simulink model "Despin_Simulink_Model"  (R2018a)
settings: Solver=VariableStepAuto  StartTime=0.0  StopTime=60  MaxStep=0.001  RelTol=1e-6  AbsTol=1e-6
values from neighbouring files (symbols this model uses):
  I_b = [151612935.5/10^9	       -12035.62/10^9        -9941.66/10^9 ... (first row only)    [Simulation_Parameters.m]
  I_single_rw = [220358.07/10^9         0               0 ... (first row only)    [Simulation_Parameters.m]
  I_st = [118601552.74/10^9	       -491524.85/10^9         95420.21/10^9 ... (first row only)    [Simulation_Parameters.m]
  m_b = 16.9927    [Simulation_Parameters.m]
  m_rw = 0.24806    [Simulation_Parameters.m]
  m_st = 9.48989    [Simulation_Parameters.m]
  R_0_to_1 = [sqrt(2)/2 0.5 0.5; -sqrt(2)/2 0.5 0.5; 0 -sqrt(2)/2 sqrt(2)/2]    [Simulation_Parameters.m]
undefined symbols (not defined in the file or in its folder): X, Y, Z
libraries: sm_lib x12, nesl_utility x10
settings Model: Creator=menel  LastModifiedBy=Menelaos
settings SolverCC: AlgebraicLoopSolver=LineSearch

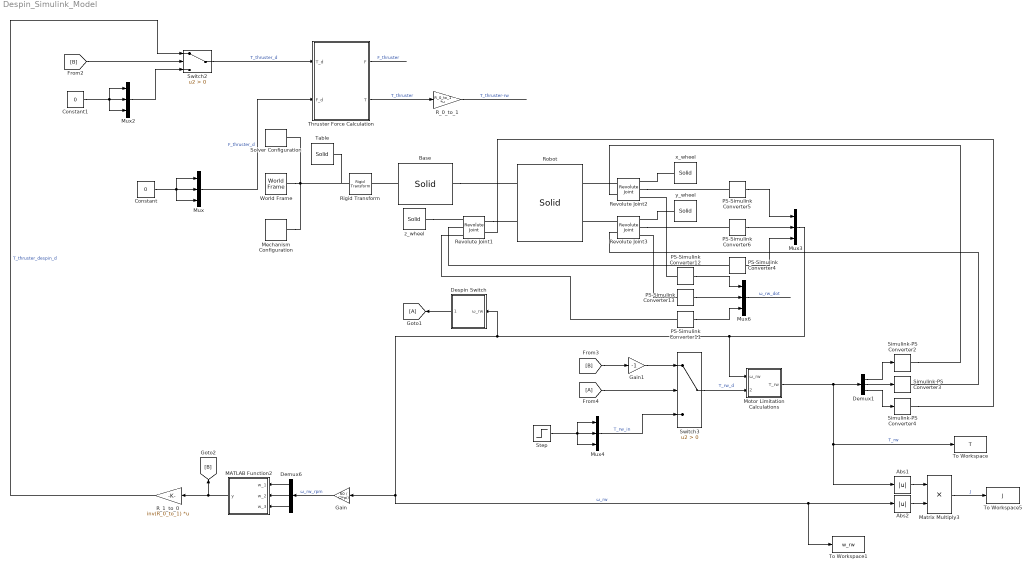
== system Despin_Simulink_Model ==
  Abs1 : Abs
  Abs2 : Abs
  Base : sm_lib/Body Elements/Solid  InertiaType=Custom  Mass=m_st  MassUnits=kg  CenterOfMass=COM_st  CenterOfMassUnits=m  MomentsOfInertia=[I_st(1,1) I_st(2,2) I_st(3,3)]  MomentsOfInertiaUnits=kg*m^2  ProductsOfInertia=[I_st(2,3) I_st(1,3) I_st(2,1)]  ProductsOfInertiaUnits=kg*m^2  DensityBased=on  Density=1000  DensityUnits=kg/m^3  DoExposeReferenceFrame=on  SerializedFrames=<Frames><Frame><Id>Frame1</Id><Value><Name>Rotation Frame</Name><Origin><Source>GeometricFeature</Source><FeatureName>spherical surface 1</FeatureName></Origin><PrimaryAxis><DefinedDirection>+Z</DefinedDirection><Source>ReferenceFrame</Source><SourceDirection>+Z</SourceDirection><FeatureName></FeatureName></PrimaryAxis><SecondaryAxis><DefinedDirection>+X</DefinedDirection><Source>ReferenceFrame</Source><SourceDirection>+X</SourceDirection><FeatureName></FeatureName></SecondaryAxis></Value></Frame></Frames>  GraphicType=FromGeometry  MarkerShape=Sphere  MarkerSize=10  GraphicVisPropType=SimpleVisualProperties  GraphicDiffuseColor=[1.0 0.2 0.2]  GraphicSpecularColor=[0.5 0.5 0.5 1.0]  GraphicAmbientColor=[0.15 0.15 0.15 1.0]  GraphicEmissiveColor=[0.0 0.0 0.0 1.0]  GraphicShininess=75  GraphicOpacity=1.0  GeometryShape=FromFile  RectangleSize=[1 1]  RectangleSizeUnits=m  BrickDimensions=[1 1 1]  BrickDimensionUnits=m  CylinderRadius=1  CylinderRadiusUnits=m  CylinderLength=1  CylinderLengthUnits=m  SphereRadius=1  SphereRadiusUnits=m  EllipsoidRadii=[1 1 1]  EllipsoidRadiiUnits=m  ExtrusionCrossSection=[1 1; -1 1; -1 -1; 1 -1]  ExtrusionCrossSectionUnits=m  ExtrusionLength=1  ExtrusionLengthUnits=m  PolygonNumSides=3  PolygonOuterRadius=1  PolygonOuterRadiusUnits=m  ExtGeomFileType=STEP  ExtGeomFileName=D:\School\Διπλωματική\Simulation\Simulation_13\Stand_6.STEP  ExtGeomFileUnits=m  RevolutionCrossSection=[1 1; 1 -1; 2 -1; 2 1]  RevolutionCrossSectionUnits=m  RevolutionExtent=Full  RevolutionAngle=180  RevolutionAngleUnits=deg
  Constant : Constant  Value=0
  Constant1 : Constant  Value=0
  Demux1 : Demux  Outputs=3
  Demux6 : Demux  Outputs=3
  Despin Switch : Subsystem
  Gain : Gain  Gain=60 / (2*pi)
  Gain1 : Gain  Gain=-1
  MATLAB Function2 : MATLAB Function  TreatAsAtomicUnit=on
  Matrix Multiply3 : Product
  Mechanism Configuration : sm_lib/Utilities/Mechanism Configuration  UniformGravity=Constant  GravityVector=[0 0 0]  GravityUnits=m/s^2  LinearizationDelta=0.001
  Motor Limitation Calculations : Subsystem
  Mux{,2..4,6} (5 alike) : Mux  Inputs=3
  PS-Simulink Converter11 : nesl_utility/PS-Simulink Converter  PhysicalDomain=network_engine_domain  SubClassName=ps_output  LeftPortType=input  RightPortType=output  PseudoPeriodic=off  Frequencies=[]  Unit=1  AffineConversion=off
  PS-Simulink Converter12 : nesl_utility/PS-Simulink Converter  PhysicalDomain=network_engine_domain  SubClassName=ps_output  LeftPortType=input  RightPortType=output  PseudoPeriodic=off  Frequencies=[]  Unit=1  AffineConversion=off
  PS-Simulink Converter13 : nesl_utility/PS-Simulink Converter  PhysicalDomain=network_engine_domain  SubClassName=ps_output  LeftPortType=input  RightPortType=output  PseudoPeriodic=off  Frequencies=[]  Unit=1  AffineConversion=off
  PS-Simulink Converter4 : nesl_utility/PS-Simulink Converter  PhysicalDomain=network_engine_domain  SubClassName=ps_output  LeftPortType=input  RightPortType=output  PseudoPeriodic=off  Frequencies=[]  Unit=rad/s  AffineConversion=off
  PS-Simulink Converter5 : nesl_utility/PS-Simulink Converter  PhysicalDomain=network_engine_domain  SubClassName=ps_output  LeftPortType=input  RightPortType=output  PseudoPeriodic=off  Frequencies=[]  Unit=rad/s  AffineConversion=off
  PS-Simulink Converter6 : nesl_utility/PS-Simulink Converter  PhysicalDomain=network_engine_domain  SubClassName=ps_output  LeftPortType=input  RightPortType=output  PseudoPeriodic=off  Frequencies=[]  Unit=rad/s  AffineConversion=off
  R_0_to_1 : Gain  Gain=R_0_to_1  Multiplication=Matrix(K*u) (u vector)
  R_1_to_0 : Gain  Gain=inv(R_0_to_1)  Multiplication=Matrix(K*u) (u vector)
  Revolute Joint1 : sm_lib/Joints/Revolute Joint  SenseConstraintForce=off  SenseConstraintForceX=off  SenseConstraintForceY=off  SenseConstraintForceZ=off  SenseConstraintTorque=off  SenseConstraintTorqueX=off  SenseConstraintTorqueY=off  SenseConstraintTorqueZ=off  SenseTotalForce=off  SenseTotalForceX=off  SenseTotalForceY=off  SenseTotalForceZ=off  SenseTotalTorque=off  SenseTotalTorqueX=off  SenseTotalTorqueY=off  SenseTotalTorqueZ=off  CompositeWrenchDir=FollowerOnBase  CompositeWrenchFrame=BaseFrame  EquilibriumPosition=0  EquilibriumPositionUnits=deg  SpringStiffness=0  SpringStiffnessUnits=N*m/deg  DampingCoefficient=0  DampingCoefficientUnits=N*m/(rad/s)  TorqueActuationMode=InputTorque  MotionActuationMode=ComputedMotion  SensePosition=off  SenseVelocity=on  SenseAcceleration=on  SenseTorqueForce=off  PositionTargetSpecify=on  PositionTargetPriority=High  PositionTargetValue=0  PositionTargetValueUnits=deg  VelocityTargetSpecify=off  VelocityTargetPriority=High  VelocityTargetValue=300  VelocityTargetValueUnits=rad/s
  Revolute Joint2 : sm_lib/Joints/Revolute Joint  SenseConstraintForce=off  SenseConstraintForceX=off  SenseConstraintForceY=off  SenseConstraintForceZ=off  SenseConstraintTorque=off  SenseConstraintTorqueX=off  SenseConstraintTorqueY=off  SenseConstraintTorqueZ=off  SenseTotalForce=off  SenseTotalForceX=off  SenseTotalForceY=off  SenseTotalForceZ=off  SenseTotalTorque=off  SenseTotalTorqueX=off  SenseTotalTorqueY=off  SenseTotalTorqueZ=off  CompositeWrenchDir=FollowerOnBase  CompositeWrenchFrame=BaseFrame  EquilibriumPosition=0  EquilibriumPositionUnits=deg  SpringStiffness=0  SpringStiffnessUnits=N*m/deg  DampingCoefficient=0  DampingCoefficientUnits=N*m/(rad/s)  TorqueActuationMode=InputTorque  MotionActuationMode=ComputedMotion  SensePosition=off  SenseVelocity=on  SenseAcceleration=on  SenseTorqueForce=off  PositionTargetSpecify=on  PositionTargetPriority=High  PositionTargetValue=0  PositionTargetValueUnits=deg  VelocityTargetSpecify=off  VelocityTargetPriority=High  VelocityTargetValue=300  VelocityTargetValueUnits=rad/s
  Revolute Joint3 : sm_lib/Joints/Revolute Joint  SenseConstraintForce=off  SenseConstraintForceX=off  SenseConstraintForceY=off  SenseConstraintForceZ=off  SenseConstraintTorque=off  SenseConstraintTorqueX=off  SenseConstraintTorqueY=off  SenseConstraintTorqueZ=off  SenseTotalForce=off  SenseTotalForceX=off  SenseTotalForceY=off  SenseTotalForceZ=off  SenseTotalTorque=off  SenseTotalTorqueX=off  SenseTotalTorqueY=off  SenseTotalTorqueZ=off  CompositeWrenchDir=FollowerOnBase  CompositeWrenchFrame=BaseFrame  EquilibriumPosition=0  EquilibriumPositionUnits=deg  SpringStiffness=0  SpringStiffnessUnits=N*m/deg  DampingCoefficient=0  DampingCoefficientUnits=N*m/(rad/s)  TorqueActuationMode=InputTorque  MotionActuationMode=ComputedMotion  SensePosition=off  SenseVelocity=on  SenseAcceleration=on  SenseTorqueForce=off  PositionTargetSpecify=on  PositionTargetPriority=High  PositionTargetValue=0  PositionTargetValueUnits=deg  VelocityTargetSpecify=off  VelocityTargetPriority=High  VelocityTargetValue=300  VelocityTargetValueUnits=rad/s
  Rigid Transform : sm_lib/Frames and Transforms/Rigid Transform  TranslationMethod=StandardAxis  TranslationStandardOffset=46  TranslationLengthUnit=mm  TranslationStandardAxis=+Z  TranslationCartesianOffset=[0 0 0]  TranslationROffset=0  TranslationROffsetUnits=m  TranslationZOffset=0  TranslationZOffsetUnits=m  TranslationThetaOffset=0  TranslationThetaOffsetUnits=deg  RotationMethod=None  RotationAngleUnits=deg  RotationStandardAxis=+Z  RotationAngle=0.0  RotationArbitraryAxis=[0 0 1]  FollAlignAxisA=+X  BaseAlignAxisA=+Y  FollAlignAxisB=+Y  BaseAlignAxisB=+Z  RotationSequenceAxes=FollowerAxes  RotationSequence=XYX  RotationSequenceAngles=[0 0 0]  RotationSequenceAnglesUnits=deg  RotationMatrix=[1 0 0; 0 1 0; 0 0 1]
  Robot : sm_lib/Body Elements/Solid  InertiaType=Custom  Mass=m_b  MassUnits=kg  CenterOfMass=COM_b  CenterOfMassUnits=m  MomentsOfInertia=[I_b(1,1) I_b(2,2) I_b(3,3)]  MomentsOfInertiaUnits=kg*m^2  ProductsOfInertia=[I_b(2,3) I_b(1,3) I_b(2,1)]  ProductsOfInertiaUnits=kg*m^2  DensityBased=off  Density=1000  DensityUnits=kg/m^3  DoExposeReferenceFrame=on  SerializedFrames=<Frames><Frame><Id>Frame1</Id><Value><Name>x wheel</Name><Origin><Source>GeometricFeature</Source><FeatureName>planar surface 30</FeatureName></Origin><PrimaryAxis><DefinedDirection>+Z</DefinedDirection><Source>GeometricFeature</Source><SourceDirection>+Z</SourceDirection><FeatureName>planar surface 30</FeatureName></PrimaryAxis><SecondaryAxis><DefinedDirection>+X</DefinedDirection><Source>ReferenceFrame</Source><SourceDirection>+X</SourceDirection><FeatureName></FeatureName></SecondaryAxis></Value></Frame><Frame><Id>Frame2</Id><Value><Name>y wheel</Name><Origin><Source>GeometricFeature</Source><FeatureName>planar surface 29</FeatureName></Origin><PrimaryAxis><DefinedDirection>+Z</DefinedDirection><Source>GeometricFeature</Source><SourceDirection>+Z</SourceDirection><FeatureName>planar surface 29</FeatureName></PrimaryAxis><SecondaryAxis><DefinedDirection>+X</DefinedDirection><Source>ReferenceFrame</Source><SourceDirection>+X</SourceDirection><FeatureName></FeatureName></SecondaryAxis></Value></Frame><Frame><Id>Frame3</Id><Value><Name>z wheel</Name><Origin><Source>GeometricFeature</Source><FeatureName>planar surface 31</FeatureName></Origin><PrimaryAxis><DefinedDirection>+Z</DefinedDirection><Source>GeometricFeature</Source><SourceDirection>+Z</SourceDirection><FeatureName>planar surface 31</FeatureName></PrimaryAxis><SecondaryAxis><DefinedDirection>+X</DefinedDirection><Source>ReferenceFrame</Source><SourceDirection>+X</SourceDirection><FeatureName></FeatureName></SecondaryAxis></Value></Frame></Frames>  GraphicType=FromGeometry  MarkerShape=Sphere  MarkerSize=10  GraphicVisPropType=SimpleVisualProperties  GraphicDiffuseColor=[0.6 0.6 1.0]  GraphicSpecularColor=[0.5 0.5 0.5 1.0]  GraphicAmbientColor=[0.15 0.15 0.15 1.0]  GraphicEmissiveColor=[0.0 0.0 0.0 1.0]  GraphicShininess=75  GraphicOpacity=1.0  GeometryShape=FromFile  RectangleSize=[1 1]  RectangleSizeUnits=m  BrickDimensions=[1 1 1]  BrickDimensionUnits=m  CylinderRadius=1  CylinderRadiusUnits=m  CylinderLength=1  CylinderLengthUnits=m  SphereRadius=1  SphereRadiusUnits=m  EllipsoidRadii=[1 1 1]  EllipsoidRadiiUnits=m  ExtrusionCrossSection=[1 1; -1 1; -1 -1; 1 -1]  ExtrusionCrossSectionUnits=m  ExtrusionLength=1  ExtrusionLengthUnits=m  PolygonNumSides=3  PolygonOuterRadius=1  PolygonOuterRadiusUnits=m  ExtGeomFileType=STEP  ExtGeomFileName=D:\School\Διπλωματική\Simulation\Simulation_13\Base_6.STEP  ExtGeomFileUnits=m  RevolutionCrossSection=[1 1; 1 -1; 2 -1; 2 1]  RevolutionCrossSectionUnits=m  RevolutionExtent=Full  RevolutionAngle=180  RevolutionAngleUnits=deg
  Simulink-PS Converter2 : nesl_utility/Simulink-PS Converter  PhysicalDomain=network_engine_domain  SubClassName=ps_input  LeftPortType=input  RightPortType=output  PseudoPeriodic=off  Frequencies=[]  NoiseDistribution=none  NoiseParameters=[]  Unit=N*m  AffineConversion=off  FilteringAndDerivatives=zero  SimscapeFilterOrder=1  InputFilterTimeConstant=0.001  UdotUserProvided=1
  Simulink-PS Converter3 : nesl_utility/Simulink-PS Converter  PhysicalDomain=network_engine_domain  SubClassName=ps_input  LeftPortType=input  RightPortType=output  PseudoPeriodic=off  Frequencies=[]  NoiseDistribution=none  NoiseParameters=[]  Unit=N*m  AffineConversion=off  FilteringAndDerivatives=zero  SimscapeFilterOrder=1  InputFilterTimeConstant=0.001  UdotUserProvided=1
  Simulink-PS Converter4 : nesl_utility/Simulink-PS Converter  PhysicalDomain=network_engine_domain  SubClassName=ps_input  LeftPortType=input  RightPortType=output  PseudoPeriodic=off  Frequencies=[]  NoiseDistribution=none  NoiseParameters=[]  Unit=N*m  AffineConversion=off  FilteringAndDerivatives=zero  SimscapeFilterOrder=1  InputFilterTimeConstant=0.001  UdotUserProvided=1
  Solver Configuration : nesl_utility/Solver Configuration  PhysicalDomain=network_engine_domain  SubClassName=solver  LeftPortType=input  RightPortType=generic  Tones=[]  Harmonics=[]  SimulateNoise=off  Profile=off  UseLocalSampling=off  EnableSwitchedLinearOptims=on  FrequencyDomain=off  UseCCode=off  RelTol=0.001  AbsTol=1e-06  MinStep=1e-09  ToWorkspace=off  RevertToSquareIcSolve=off  NumHomotopyIterations=100  PhasorMode=off  PhasorModeNumHarmonics=1  DoDC=off  ResidualTolerance=1e-09  UseLocalSolver=off  LocalSolverChoice=NE_BACKWARD_EULER_ADVANCER  LocalSolverSampleTime=0.001  DoFixedCost=off  MaxNonlinIter=3  MaxModeIter=2  LinearAlgebra=Sparse  EquationFormulation=NE_TIME_EF  DelaysMemoryBudget=1024  AutomaticFiltering=on  FilteringTimeConstant=0.001
  Step : Step  Time=30  Before=0.01  After=0  SampleTime=0
  Switch2 : Switch  Criteria=u2 > Threshold
  Switch3 : Switch  Criteria=u2 > Threshold
  Table : sm_lib/Body Elements/Solid  InertiaType=CalculateFromGeometry  Mass=1  MassUnits=kg  CenterOfMass=[0 0 0]  CenterOfMassUnits=m  MomentsOfInertia=[1 1 1]  MomentsOfInertiaUnits=kg*m^2  ProductsOfInertia=[0 0 0]  ProductsOfInertiaUnits=kg*m^2  DensityBased=on  Density=1000  DensityUnits=kg/m^3  DoExposeReferenceFrame=on  SerializedFrames=<Frames/>  GraphicType=FromGeometry  MarkerShape=Sphere  MarkerSize=10  GraphicVisPropType=SimpleVisualProperties  GraphicDiffuseColor=[0.5 0.5 0.5]  GraphicSpecularColor=[0.5 0.5 0.5 1.0]  GraphicAmbientColor=[0.15 0.15 0.15 1.0]  GraphicEmissiveColor=[0.0 0.0 0.0 1.0]  GraphicShininess=75  GraphicOpacity=1.0  GeometryShape=FromFile  RectangleSize=[1 1]  RectangleSizeUnits=m  BrickDimensions=[1 1 1]  BrickDimensionUnits=m  CylinderRadius=1  CylinderRadiusUnits=m  CylinderLength=1  CylinderLengthUnits=m  SphereRadius=1  SphereRadiusUnits=m  EllipsoidRadii=[1 1 1]  EllipsoidRadiiUnits=m  ExtrusionCrossSection=[1 1; -1 1; -1 -1; 1 -1]  ExtrusionCrossSectionUnits=m  ExtrusionLength=1  ExtrusionLengthUnits=m  PolygonNumSides=3  PolygonOuterRadius=1  PolygonOuterRadiusUnits=m  ExtGeomFileType=STEP  ExtGeomFileName=D:\School\Διπλωματική\Simulation\Simulation_13\Table.STEP  ExtGeomFileUnits=m  RevolutionCrossSection=[1 1; 1 -1; 2 -1; 2 1]  RevolutionCrossSectionUnits=m  RevolutionExtent=Full  RevolutionAngle=180  RevolutionAngleUnits=deg
  Thruster Force Calculation : Subsystem
  To Workspace : ToWorkspace  VariableName=T  SampleTime=-1
  To Workspace1 : ToWorkspace  VariableName=w_rw  SampleTime=-1
  To Workspace5 : ToWorkspace  VariableName=J  SampleTime=-1
  World Frame : sm_lib/Frames and Transforms/World Frame
  x_wheel : sm_lib/Body Elements/Solid  InertiaType=Custom  Mass=m_rw  MassUnits=kg  CenterOfMass=COM_rw  CenterOfMassUnits=m  MomentsOfInertia=[I_single_rw(1,1) I_single_rw(2,2) I_single_rw(3,3)]  MomentsOfInertiaUnits=kg*m^2  ProductsOfInertia=[I_single_rw(2,3) I_single_rw(1,3) I_single_rw(2,1)]  ProductsOfInertiaUnits=kg*m^2  DensityBased=off  Density=1000  DensityUnits=kg/m^3  DoExposeReferenceFrame=off  SerializedFrames=<Frames><Frame><Id>Frame1</Id><Value><Name>R</Name><Origin><Source>GeometricFeature</Source><FeatureName>planar surface 2</FeatureName></Origin><PrimaryAxis><DefinedDirection>+Z</DefinedDirection><Source>ReferenceFrame</Source><SourceDirection>+Z</SourceDirection><FeatureName></FeatureName></PrimaryAxis><SecondaryAxis><DefinedDirection>+X</DefinedDirection><Source>ReferenceFrame</Source><SourceDirection>+X</SourceDirection><FeatureName></FeatureName></SecondaryAxis></Value></Frame></Frames>  GraphicType=FromGeometry  MarkerShape=Sphere  MarkerSize=10  GraphicVisPropType=SimpleVisualProperties  GraphicDiffuseColor=[1.0 0.2 0.2]  GraphicSpecularColor=[0.5 0.5 0.5 1.0]  GraphicAmbientColor=[0.15 0.15 0.15 1.0]  GraphicEmissiveColor=[0.0 0.0 0.0 1.0]  GraphicShininess=75  GraphicOpacity=1.0  GeometryShape=FromFile  RectangleSize=[1 1]  RectangleSizeUnits=m  BrickDimensions=[1 1 1]  BrickDimensionUnits=m  CylinderRadius=1  CylinderRadiusUnits=m  CylinderLength=1  CylinderLengthUnits=m  SphereRadius=1  SphereRadiusUnits=m  EllipsoidRadii=[1 1 1]  EllipsoidRadiiUnits=m  ExtrusionCrossSection=[1 1; -1 1; -1 -1; 1 -1]  ExtrusionCrossSectionUnits=m  ExtrusionLength=1  ExtrusionLengthUnits=m  PolygonNumSides=3  PolygonOuterRadius=1  PolygonOuterRadiusUnits=m  ExtGeomFileType=STEP  ExtGeomFileName=D:\School\Διπλωματική\Simulation\Simulation_13\Reaction_Wheel_6.STEP  ExtGeomFileUnits=m  RevolutionCrossSection=[1 1; 1 -1; 2 -1; 2 1]  RevolutionCrossSectionUnits=m  RevolutionExtent=Full  RevolutionAngle=180  RevolutionAngleUnits=deg
  y_wheel : sm_lib/Body Elements/Solid  InertiaType=Custom  Mass=m_rw  MassUnits=kg  CenterOfMass=COM_rw  CenterOfMassUnits=m  MomentsOfInertia=[I_single_rw(1,1) I_single_rw(2,2) I_single_rw(3,3)]  MomentsOfInertiaUnits=kg*m^2  ProductsOfInertia=[I_single_rw(2,3) I_single_rw(1,3) I_single_rw(2,1)]  ProductsOfInertiaUnits=kg*m^2  DensityBased=off  Density=1000  DensityUnits=kg/m^3  DoExposeReferenceFrame=off  SerializedFrames=<Frames><Frame><Id>Frame1</Id><Value><Name>R</Name><Origin><Source>GeometricFeature</Source><FeatureName>planar surface 2</FeatureName></Origin><PrimaryAxis><DefinedDirection>+Z</DefinedDirection><Source>ReferenceFrame</Source><SourceDirection>+Z</SourceDirection><FeatureName></FeatureName></PrimaryAxis><SecondaryAxis><DefinedDirection>+X</DefinedDirection><Source>ReferenceFrame</Source><SourceDirection>+X</SourceDirection><FeatureName></FeatureName></SecondaryAxis></Value></Frame></Frames>  GraphicType=FromGeometry  MarkerShape=Sphere  MarkerSize=10  GraphicVisPropType=SimpleVisualProperties  GraphicDiffuseColor=[1.0 0.2 0.2]  GraphicSpecularColor=[0.5 0.5 0.5 1.0]  GraphicAmbientColor=[0.15 0.15 0.15 1.0]  GraphicEmissiveColor=[0.0 0.0 0.0 1.0]  GraphicShininess=75  GraphicOpacity=1.0  GeometryShape=FromFile  RectangleSize=[1 1]  RectangleSizeUnits=m  BrickDimensions=[1 1 1]  BrickDimensionUnits=m  CylinderRadius=1  CylinderRadiusUnits=m  CylinderLength=1  CylinderLengthUnits=m  SphereRadius=1  SphereRadiusUnits=m  EllipsoidRadii=[1 1 1]  EllipsoidRadiiUnits=m  ExtrusionCrossSection=[1 1; -1 1; -1 -1; 1 -1]  ExtrusionCrossSectionUnits=m  ExtrusionLength=1  ExtrusionLengthUnits=m  PolygonNumSides=3  PolygonOuterRadius=1  PolygonOuterRadiusUnits=m  ExtGeomFileType=STEP  ExtGeomFileName=D:\School\Διπλωματική\Simulation\Simulation_13\Reaction_Wheel_6.STEP  ExtGeomFileUnits=m  RevolutionCrossSection=[1 1; 1 -1; 2 -1; 2 1]  RevolutionCrossSectionUnits=m  RevolutionExtent=Full  RevolutionAngle=180  RevolutionAngleUnits=deg
  z_wheel : sm_lib/Body Elements/Solid  InertiaType=Custom  Mass=m_rw  MassUnits=kg  CenterOfMass=COM_rw  CenterOfMassUnits=m  MomentsOfInertia=[I_single_rw(1,1) I_single_rw(2,2) I_single_rw(3,3)]  MomentsOfInertiaUnits=kg*m^2  ProductsOfInertia=[I_single_rw(2,3) I_single_rw(1,3) I_single_rw(2,1)]  ProductsOfInertiaUnits=kg*m^2  DensityBased=off  Density=1000  DensityUnits=kg/m^3  DoExposeReferenceFrame=off  SerializedFrames=<Frames><Frame><Id>Frame1</Id><Value><Name>R</Name><Origin><Source>GeometricFeature</Source><FeatureName>planar surface 2</FeatureName></Origin><PrimaryAxis><DefinedDirection>+Z</DefinedDirection><Source>ReferenceFrame</Source><SourceDirection>+Z</SourceDirection><FeatureName></FeatureName></PrimaryAxis><SecondaryAxis><DefinedDirection>+X</DefinedDirection><Source>ReferenceFrame</Source><SourceDirection>+X</SourceDirection><FeatureName></FeatureName></SecondaryAxis></Value></Frame></Frames>  GraphicType=FromGeometry  MarkerShape=Sphere  MarkerSize=10  GraphicVisPropType=SimpleVisualProperties  GraphicDiffuseColor=[1.0 0.2 0.2]  GraphicSpecularColor=[0.5 0.5 0.5 1.0]  GraphicAmbientColor=[0.15 0.15 0.15 1.0]  GraphicEmissiveColor=[0.0 0.0 0.0 1.0]  GraphicShininess=75  GraphicOpacity=1.0  GeometryShape=FromFile  RectangleSize=[1 1]  RectangleSizeUnits=m  BrickDimensions=[1 1 1]  BrickDimensionUnits=m  CylinderRadius=1  CylinderRadiusUnits=m  CylinderLength=1  CylinderLengthUnits=m  SphereRadius=1  SphereRadiusUnits=m  EllipsoidRadii=[1 1 1]  EllipsoidRadiiUnits=m  ExtrusionCrossSection=[1 1; -1 1; -1 -1; 1 -1]  ExtrusionCrossSectionUnits=m  ExtrusionLength=1  ExtrusionLengthUnits=m  PolygonNumSides=3  PolygonOuterRadius=1  PolygonOuterRadiusUnits=m  ExtGeomFileType=STEP  ExtGeomFileName=D:\School\Διπλωματική\Simulation\Simulation_13\Reaction_Wheel_6.STEP  ExtGeomFileUnits=m  RevolutionCrossSection=[1 1; 1 -1; 2 -1; 2 1]  RevolutionCrossSectionUnits=m  RevolutionExtent=Full  RevolutionAngle=180  RevolutionAngleUnits=deg
  wires:
  Mux/1 -> Thruster Force Calculation/2(F_d)  "F_thruster_d"
  Thruster Force Calculation/1(F) -> ?  "F_thruster"
  Thruster Force Calculation/2(T) -> R_0_to_1/1  "T_thruster"
  PS-Simulink Converter6/1 -> Mux3/2
  PS-Simulink Converter5/1 -> Mux3/1
  PS-Simulink Converter4/1 -> Mux3/3
  Mux3/1 -> Motor Limitation Calculations/1(ω_rw), To Workspace1/1, Abs2/1, Gain/1, Despin Switch/1(ω_rw)  "ω_rw"
  Demux1/2 -> Simulink-PS Converter3/1
  Demux1/3 -> Simulink-PS Converter4/1
  Demux1/1 -> Simulink-PS Converter2/1
  Mux6/1 -> ?  "ω_rw_dot"
  Constant/1 -> Mux/3, Mux/1, Mux/2
  PS-Simulink Converter12/1 -> Mux6/1
  PS-Simulink Converter13/1 -> Mux6/2
  PS-Simulink Converter11/1 -> Mux6/3
  Gain/1 -> Demux6/1  "ω_rw_rpm"
  Demux6/3 -> MATLAB Function2/3(w_3)
  Demux6/2 -> MATLAB Function2/2(w_2)
  Demux6/1 -> MATLAB Function2/1(w_1)
  MATLAB Function2/1(y) -> [B], R_1_to_0/1
  [B] -> Switch2/2
  Switch2/1 -> Thruster Force Calculation/1(T_d)  "T_thruster_d"
  Mux2/1 -> Switch2/3
  Constant1/1 -> Mux2/3, Mux2/1, Mux2/2
  R_0_to_1/1 -> ?  "T_thruster-rw"
  R_1_to_0/1 -> Switch2/1  "T_thruster_despin_d"
  [A] -> Switch3/2
  Mux4/1 -> Switch3/3  "T_rw_in"
  [B] -> Gain1/1
  Despin Switch/1(signal) -> [A]
  Step/1 -> Mux4/3, Mux4/1, Mux4/2
  Motor Limitation Calculations/1(T_rw) -> To Workspace/1, Abs1/1, Demux1/1  "T_rw"
  Switch3/1 -> Motor Limitation Calculations/2(T_rw_d)  "T_rw_d"
  Gain1/1 -> Switch3/1
  Abs2/1 -> Matrix Multiply3/2
  Abs1/1 -> Matrix Multiply3/1
  Matrix Multiply3/1 -> To Workspace5/1  "J"
  connections:
  World Frame/RConn1 -- Mechanism Configuration/RConn1 -- Table/RConn1 -- Rigid Transform/LConn1 -- Solver Configuration/RConn1
  Base/RConn1 -- Rigid Transform/RConn1
  Revolute Joint1/LConn1 -- Robot/RConn2
  z_wheel/LConn1 -- Revolute Joint1/RConn1
  Revolute Joint2/LConn1 -- Robot/LConn1
  Revolute Joint3/LConn1 -- Robot/LConn2
  x_wheel/LConn1 -- Revolute Joint2/RConn1
  y_wheel/LConn1 -- Revolute Joint3/RConn1
  Revolute Joint2/RConn2 -- PS-Simulink Converter5/LConn1
  Revolute Joint3/RConn2 -- PS-Simulink Converter6/LConn1
  PS-Simulink Converter4/LConn1 -- Revolute Joint1/RConn2
  Simulink-PS Converter2/RConn1 -- Revolute Joint2/LConn2
  Simulink-PS Converter3/RConn1 -- Revolute Joint3/LConn2
  Simulink-PS Converter4/RConn1 -- Revolute Joint1/LConn2
  PS-Simulink Converter12/LConn1 -- Revolute Joint2/RConn3
  PS-Simulink Converter13/LConn1 -- Revolute Joint3/RConn3
  PS-Simulink Converter11/LConn1 -- Revolute Joint1/RConn3
  Base/LConn1 -- Robot/RConn1

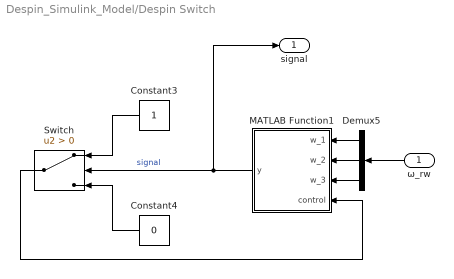
== system Despin_Simulink_Model/Despin Switch ==
  ω_rw : Inport
  Constant3 : Constant
  Constant4 : Constant  Value=0
  Demux5 : Demux  Outputs=3
  MATLAB Function1 : MATLAB Function  TreatAsAtomicUnit=on
  Switch : Switch  Criteria=u2 > Threshold
  signal : Outport
  wires:
  ω_rw/1 -> Demux5/1
  Demux5/3 -> MATLAB Function1/3(w_3)
  Demux5/1 -> MATLAB Function1/1(w_1)
  Constant3/1 -> Switch/1
  Switch/1 -> MATLAB Function1/4(control)
  MATLAB Function1/1(y) -> signal/1, Switch/2  "signal"
  Constant4/1 -> Switch/3
  Demux5/2 -> MATLAB Function1/2(w_2)

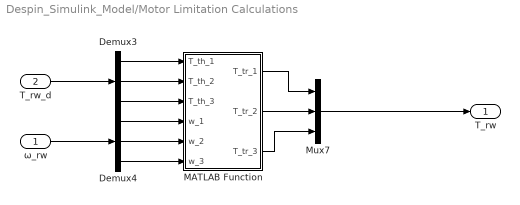
== system Despin_Simulink_Model/Motor Limitation Calculations ==
  ω_rw : Inport
  T_rw_d : Inport  Port=2
  Demux3 : Demux  Outputs=3
  Demux4 : Demux  Outputs=3
  MATLAB Function : MATLAB Function  TreatAsAtomicUnit=on
  Mux7 : Mux  Inputs=3
  T_rw : Outport
  wires:
  Demux3/1 -> MATLAB Function/1(T_th_1)
  Demux4/1 -> MATLAB Function/4(w_1)
  Demux3/3 -> MATLAB Function/3(T_th_3)
  Demux4/2 -> MATLAB Function/5(w_2)
  MATLAB Function/3(T_tr_3) -> Mux7/3
  Demux3/2 -> MATLAB Function/2(T_th_2)
  MATLAB Function/2(T_tr_2) -> Mux7/2
  MATLAB Function/1(T_tr_1) -> Mux7/1
  Demux4/3 -> MATLAB Function/6(w_3)
  ω_rw/1 -> Demux4/1
  Mux7/1 -> T_rw/1
  T_rw_d/1 -> Demux3/1

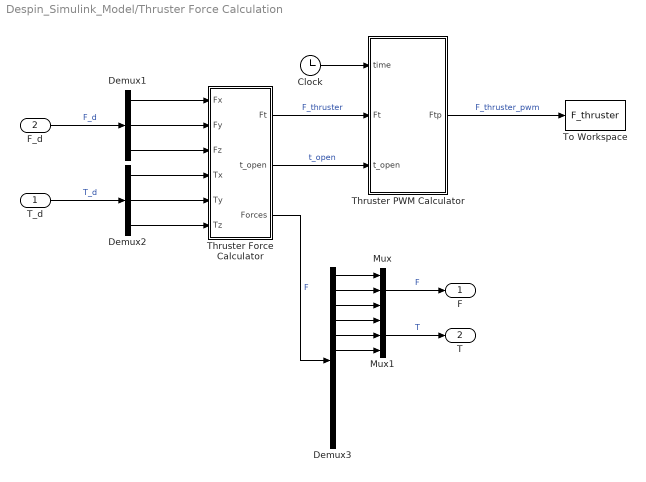
== system Despin_Simulink_Model/Thruster Force Calculation ==
  T_d : Inport
  F_d : Inport  Port=2
  Clock : Clock
  Demux1 : Demux  Outputs=3
  Demux2 : Demux  Outputs=3
  Demux3 : Demux  Outputs=12
  Mux : Mux  Inputs=3
  Mux1 : Mux  Inputs=3
  Thruster Force Calculator : MATLAB Function  TreatAsAtomicUnit=on
  Thruster PWM Calculator : MATLAB Function  TreatAsAtomicUnit=on
  To Workspace : ToWorkspace  VariableName=F_thruster  SampleTime=-1
  F : Outport
  T : Outport  Port=2
  wires:
  Demux2/3 -> Thruster Force Calculator/6(Tz)
  Demux1/3 -> Thruster Force Calculator/3(Fz)
  Demux2/1 -> Thruster Force Calculator/4(Tx)
  Demux1/2 -> Thruster Force Calculator/2(Fy)
  Demux1/1 -> Thruster Force Calculator/1(Fx)
  Demux2/2 -> Thruster Force Calculator/5(Ty)
  T_d/1 -> Demux2/1  "T_d"
  F_d/1 -> Demux1/1  "F_d"
  Thruster Force Calculator/2(t_open) -> Thruster PWM Calculator/3(t_open)  "t_open"
  Thruster Force Calculator/1(Ft) -> Thruster PWM Calculator/2(Ft)  "F_thruster"
  Clock/1 -> Thruster PWM Calculator/1(time)
  Thruster PWM Calculator/1(Ftp) -> To Workspace/1  "F_thruster_pwm"
  Thruster Force Calculator/3(Forces) -> Demux3/1  "F"
  Demux3/1 -> Mux/1
  Demux3/2 -> Mux/2
  Demux3/3 -> Mux/3
  Demux3/4 -> Mux1/1
  Demux3/5 -> Mux1/2
  Demux3/6 -> Mux1/3
  Mux/1 -> F/1  "F"
  Mux1/1 -> T/1  "T"

== matlab function Despin_Simulink_Model/Thruster Force Calculation/Thruster Force Calculator ==
  data: Ft output; t_open output; Fx input; Fy input; Fz input; Tx input; Ty input; Tz input; Forces output
function [Ft,t_open,Forces]= fcn(Fx,Fy,Fz,Tx,Ty,Tz)

f = [Fx;Fy;Fz;Tx;Ty;Tz];

d = 0.2335;
T = 0.1;

A = [-1  cosd(60)   cosd(60)  0        0            0;
      0  sind(60)  -sind(60)  0        0            0;
      0     0          0      1        1            1;
      0     0          0      d  -d*cosd(30)  -d*cosd(30);
      0     0          0      0  -d*sind(30)   d*sind(30);
      d     d          d      0        0            0   ];

Ft_d = inv(A)*f;

Ft = [0;0;0;0;0;0;0;0;0;0;0;0];
t_open = [0;0;0;0;0;0;0;0;0;0;0;0];

if Ft_d(1) == 0
    
    Ft(1) = 0;
    Ft(2) = 0;
    t_open(1) = 0;
    t_open(2) = 0;
    
elseif Ft_d(1) > 0
    
    Ft(1) = 1;
    Ft(2) = 0;
    t_open(1) = abs(Ft_d(1)*T);
    t_open(2) = 0;
    
else
    
    Ft(1) = 0;
    Ft(2) = 1;
    t_open(1) = 0;
    t_open(2) = abs(Ft_d(1)*T);
    
end

%%%%%%%%%%%%%%%%%%%%%%%%%%%%%%%%%%%%%%%%%%%%%%%%%%%%%%%%%%%%%%

if Ft_d(2) == 0
    
    Ft(3) = 0;
    Ft(4) = 0;
    t_open(3) = 0;
    t_open(4) = 0;
    
elseif Ft_d(2) > 0
    
    Ft(3) = 1;
    Ft(4) = 0;
    t_open(3) = abs(Ft_d(2)*T);
    t_open(4) = 0;
    
else
    
    Ft(3) = 0;
    Ft(4) = 1;
    t_open(3) = 0;
    t_open(4) = abs(Ft_d(2)*T);
    
end

%%%%%%%%%%%%%%%%%%%%%%%%%%%%%%%%%%%%%%%%%%%%%%%%%%%%%%%%%%%%%%

if Ft_d(3) == 0
    
    Ft(5) = 0;
    Ft(6) = 0;
    t_open(5) = 0;
    t_open(6) = 0;
    
elseif Ft_d(3) > 0
    
    Ft(5) = 1;
    Ft(6) = 0;
    t_open(5) = abs(Ft_d(3)*T);
    t_open(6) = 0;
    
else
    
    Ft(5) = 0;
    Ft(6) = 1;
    t_open(5) = 0;
    t_open(6) = abs(Ft_d(3)*T);
    
end

%%%%%%%%%%%%%%%%%%%%%%%%%%%%%%%%%%%%%%%%%%%%%%%%%%%%%%%%%%%%%%

if Ft_d(4) == 0
    
    Ft(7) = 0;
    Ft(8) = 0;
    t_open(7) = 0;
    t_open(8) = 0;
    
elseif Ft_d(4) > 0
    
    Ft(7) = 1;
    Ft(8) = 0;
    t_open(7) = abs(Ft_d(4)*T);
    t_open(8) = 0;
    
else
    
    Ft(7) = 0;
    Ft(8) = 1;
    t_open(7) = 0;
    t_open(8) = abs(Ft_d(4)*T);
    
end

%%%%%%%%%%%%%%%%%%%%%%%%%%%%%%%%%%%%%%%%%%%%%%%%%%%%%%%%%%%%%%

if Ft_d(5) == 0
    
    Ft(9) = 0;
    Ft(10) = 0;
    t_open(9) = 0;
    t_open(10) = 0;
    
elseif Ft_d(5) > 0
    
    Ft(9) = 1;
    Ft(10) = 0;
    t_open(9) = abs(Ft_d(5)*T);
    t_open(10) = 0;
    
else
    
    Ft(9) = 0;
    Ft(10) = 1;
    t_open(9) = 0;
    t_open(10) = abs(Ft_d(5)*T);
    
end

%%%%%%%%%%%%%%%%%%%%%%%%%%%%%%%%%%%%%%%%%%%%%%%%%%%%%%%%%%%%%%

if Ft_d(6) == 0
    
    Ft(11) = 0;
    Ft(12) = 0;
    t_open(11) = 0;
    t_open(12) = 0;
    
elseif Ft_d(6) > 0
    
    Ft(11) = 1;
    Ft(12) = 0;
    t_open(11) = abs(Ft_d(6)*T);
    t_open(12) = 0;
    
else
    
    Ft(11) = 0;
    Ft(12) = 1;
    t_open(11) = 0;
    t_open(12) = abs(Ft_d(6)*T);
    
end

for i = 1:6
    if Ft_d(i) > 1
        
        Ft_d(i) = 1;
        
    elseif Ft_d(i) < -1
        
        Ft_d(i) = -1;
        
    end
end
 
FT = A * Ft_d;

Forces = [FT(1);FT(2);FT(3);FT(4);FT(5);FT(6);0;0;0;0;0;0];

== matlab function Despin_Simulink_Model/Thruster Force Calculation/Thruster PWM Calculator ==
  data: time input; Ft input; Ftp output; t_open input
function Ftp = fcn(time,Ft,t_open)

P = 0.1;

t = time - fix(time/P)*P;
Ftp = [0;0;0;0;0;0;0;0;0;0;0;0];

for i = 1:12
    if t <= t_open(i)
        Ftp(i) = Ft(i);
    else
        Ftp(i) = 0;
    end
end

== matlab function Despin_Simulink_Model/Despin Switch/MATLAB Function1 ==
  data: w_1 input; y output; w_2 input; w_3 input; control input
function y = fcn(w_1,w_2,w_3,control)

w_1 = w_1 * 60 / (2*pi);
w_2 = w_2 * 60 / (2*pi);
w_3 = w_3 * 60 / (2*pi);

if control == 0
    y = 0;
else
    if (abs(w_1) <= 50) && (abs(w_2) <= 50) && (abs(w_3) <= 50)
        y = 0;
    else
        y = 1;
    end
end

if (abs(w_1) >= 6000) || (abs(w_2) >= 6000) || (abs(w_3) >= 6000)
    y = 1;
end

== matlab function Despin_Simulink_Model/MATLAB Function2 ==
  data: w_1 input; y output; w_2 input; w_3 input
function y = fcn(w_1,w_2,w_3)

T_d = [0;0;0];
t_disp = 1;
max_rpm = max([abs(w_1) abs(w_2) abs(w_3)]);
a_disp = (max_rpm - 50) / t_disp;
I_rw_z = 418129.72/10^9;
T_disp = I_rw_z * a_disp;
% 0.0911;

if abs(w_1) > 50
    if w_1 > 0
        T_d(1) = T_disp;
    else
        T_d(1) = -T_disp;
    end
else
    T_d(1) = 0;
end

if abs(w_2) > 50
    if w_2 > 0
        T_d(2) = T_disp;
    else
        T_d(2) = -T_disp;
    end
else
    T_d(2) = 0;
end

if abs(w_3) > 50
    if w_3 > 0
        T_d(3) = T_disp;
    else
        T_d(3) = -T_disp;
    end
else
    T_d(3) = 0;
end

y = T_d;

== matlab function Despin_Simulink_Model/Motor Limitation Calculations/MATLAB Function ==
  data: T_th_1 input; T_tr_1 output; T_th_2 input; T_th_3 input; w_1 input; w_2 input; w_3 input; T_tr_2 output; T_tr_3 output
function [T_tr_1,T_tr_2,T_tr_3] = fcn(T_th_1,T_th_2,T_th_3,w_1,w_2,w_3)

T_max = 3 * 0.0911;
T_max_1 = T_max;
T_max_2 = T_max;
T_max_3 = T_max;
T_max_c = T_max;

if abs(w_1) > 0
    if (abs(w_1) * abs(T_th_1)) >= 50
        T_max_1 = 50/abs(w_1);
    end
end

w_1 = w_1 * 60 / (2*pi);

if abs(w_1) >= 10000
    T_max_2 = 0;
end

if (abs(w_1)/265 + abs(T_th_1)*6920/265) >= 29.6
    T_max_3 = 265*29.6/6920 - abs(w_1)/6920;
end

if T_max_c > T_max_1
    T_max_c = T_max_1;
end
if T_max_c > T_max_2
    T_max_c = T_max_2;
end
if T_max_c > T_max_3
    T_max_c = T_max_3;
end

test_1 = T_max_c;

if abs(T_th_1) > T_max_c
    if T_th_1 >= 0
        T_tr_1 = T_max_c;
    else
        T_tr_1 = -T_max_c;
    end
else
    T_tr_1 = T_th_1;
end

%%%%%%%%%%%%%%%%%%%%%%%%%%%%%%%%%%%%%%%%%%%%%%%%%%%%%%%%%%%%%%%%%%%%

T_max_1 = T_max;
T_max_2 = T_max;
T_max_3 = T_max;
T_max_c = T_max;

if abs(w_2) > 0
    if (abs(w_2) * abs(T_th_2)) >= 50
        T_max_1 = 50/abs(w_2);
    end
end

w_2 = w_2 * 60 / (2*pi);

if abs(w_2) >= 10000
    T_max_2 = 0;
end

if (abs(w_2)/265 + abs(T_th_2)*6920/265) >= 29.6
    T_max_3 = 265*29.6/6920 - abs(w_2)/6920;
end

if T_max_c > T_max_1
    T_max_c = T_max_1;
end
if T_max_c > T_max_2
    T_max_c = T_max_2;
end
if T_max_c > T_max_3
    T_max_c = T_max_3;
end

test_2 = T_max_c;

if abs(T_th_2) > T_max_c
    if T_th_2 >= 0
        T_tr_2 = T_max_c;
    else
        T_tr_2 = -T_max_c;
    end
else
    T_tr_2 = T_th_2;
end

%%%%%%%%%%%%%%%%%%%%%%%%%%%%%%%%%%%%%%%%%%%%%%%%%%%%%%%%%%%%%%%%%%%%

T_max_1 = T_max;
T_max_2 = T_max;
T_max_3 = T_max;
T_max_c = T_max;

if abs(w_3) > 0
    if (abs(w_3) * abs(T_th_3)) >= 29.6
        T_max_1 = 50/abs(w_3);
    end
end

w_3 = w_3 * 60 / (2*pi);

if abs(w_3) >= 10000
    T_max_2 = 0;
end

if (abs(w_3)/265 + abs(T_th_3)*6920/265) >= 60
    T_max_3 = 265*29.6/6920 - abs(w_3)/6920;
end

if T_max_c > T_max_1
    T_max_c = T_max_1;
end
if T_max_c > T_max_2
    T_max_c = T_max_2;
end
if T_max_c > T_max_3
    T_max_c = T_max_3;
end

test_3 = T_max_c;

if abs(T_th_3) > T_max_c
    if T_th_3 >= 0
        T_tr_3 = T_max_c;
    else
        T_tr_3 = -T_max_c;
    end
else
    T_tr_3 = T_th_3;
end
